simulink model "MotorModelZJChen"  (R2020b)
settings: Solver=VariableStepAuto  StartTime=0.0  StopTime=10.0  RelTol=1e-3  EnableMultiTasking=on
undefined symbols (not defined in the file): Aero, Initial, Motor, Uav
libraries: QuaternionLibrary x1
settings Model: Creator=jban039  LastModifiedBy=jban039
settings DataIOCC: LimitDataPoints=on
settings OptimizationCC: LifeSpan=inf
settings DebuggingCC: AllowSymbolicDim=off  SFUnexpectedBacktrackingDiag=warning  SFNoUnconditionalDefaultTransitionDiag=warning  SFExecutionAtInitializationDiag=none  ArithmeticOperatorsInVariantConditions=warning
settings ModelReferenceCC: PropagateSignalLabelsOutOfModel=off
settings SFSimCC: SimUseLocalCustomCode=off  CustomCodeUndefinedFunction=UseInterfaceOnly
settings RTWCC: RTWUseLocalCustomCode=off
settings CodeAppCC: StateflowObjectComments=on
settings GRTTargetCC: TargetLangStandard=C89/C90 (ANSI)
settings ConfigComp: CovMetricSettings=dw  CovSaveCumulativeToWorkspaceVar=on  CovSaveSingleToWorkspaceVar=on  CovExternalEMLEnable=off

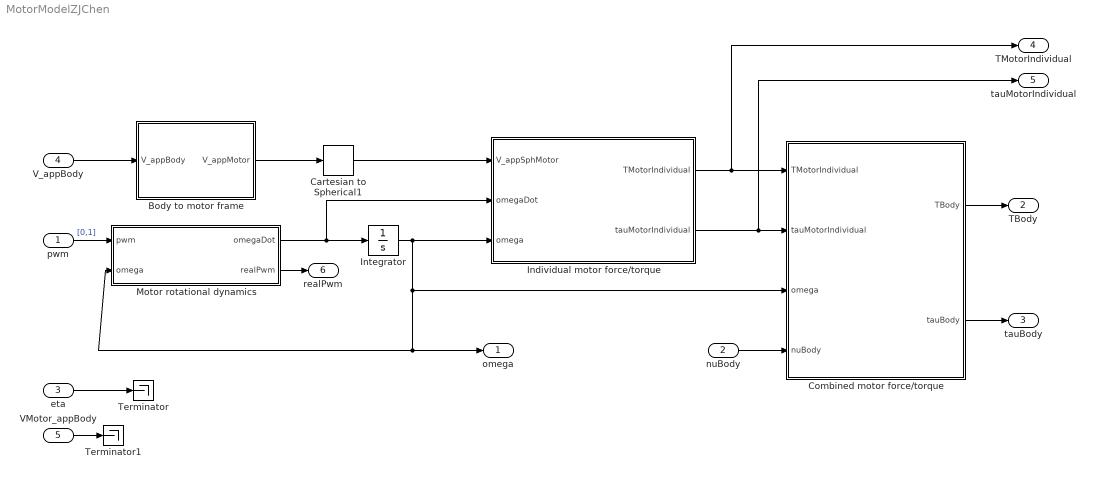
== system MotorModelZJChen ==
  pwm : Inport  PortDimensions=Uav.N_ROTORS
  nuBody : Inport  Port=2  Unit=rad/s  PortDimensions=3
  eta : Inport  Port=3  Unit=rad  PortDimensions=3
  V_appBody : Inport  Port=4  Unit=m/s  PortDimensions=3
  VMotor_appBody : Inport  Port=5  Unit=m/s  PortDimensions=[3,Uav.N_ROTORS]
  Body to motor frame : MATLAB Function  TreatAsAtomicUnit=on
  Cartesian to Spherical1 : QuaternionLibrary/Cartesian to Spherical
  Combined motor force/torque : MATLAB Function  TreatAsAtomicUnit=on
  Individual motor force/torque : MATLAB Function  TreatAsAtomicUnit=on
  Integrator : Integrator  InitialCondition=Initial.OMEGA  LimitOutput=on  LowerSaturationLimit=zeros(size(Initial.OMEGA))  ContinuousStateAttributes='omega'
  Motor rotational dynamics : MATLAB Function  TreatAsAtomicUnit=on
  Terminator : Terminator
  Terminator1 : Terminator
  omega : Outport  Unit=rad/s  VectorParamsAs1DForOutWhenUnconnected=off
  TBody : Outport  Port=2  Unit=N  VectorParamsAs1DForOutWhenUnconnected=off
  tauBody : Outport  Port=3  Unit=N*m  VectorParamsAs1DForOutWhenUnconnected=off
  TMotorIndividual : Outport  Port=4  Unit=N  PortDimensions=[3,Uav.N_ROTORS]  VectorParamsAs1DForOutWhenUnconnected=off
  tauMotorIndividual : Outport  Port=5  Unit=N  PortDimensions=[3,Uav.N_ROTORS]  VectorParamsAs1DForOutWhenUnconnected=off
  realPwm : Outport  Port=6  VectorParamsAs1DForOutWhenUnconnected=off
  wires:
  Combined motor force/torque/2(tauBody) -> tauBody/1
  Combined motor force/torque/1(TBody) -> TBody/1
  pwm/1 -> Motor rotational dynamics/1(pwm)  "[0,1]"
  eta/1 -> Terminator/1
  V_appBody/1 -> Body to motor frame/1(V_appBody)
  Individual motor force/torque/2(tauMotorIndividual) -> tauMotorIndividual/1, Combined motor force/torque/2(tauMotorIndividual)
  nuBody/1 -> Combined motor force/torque/4(nuBody)
  Individual motor force/torque/1(TMotorIndividual) -> TMotorIndividual/1, Combined motor force/torque/1(TMotorIndividual)
  Motor rotational dynamics/1(omegaDot) -> Individual motor force/torque/2(omegaDot), Integrator/1
  Integrator/1 -> Individual motor force/torque/3(omega), Combined motor force/torque/3(omega), Motor rotational dynamics/2(omega), omega/1
  Motor rotational dynamics/2(realPwm) -> realPwm/1
  VMotor_appBody/1 -> Terminator1/1
  Body to motor frame/1(V_appMotor) -> Cartesian to Spherical1/1
  Cartesian to Spherical1/1 -> Individual motor force/torque/1(V_appSphMotor)

== matlab function MotorModelZJChen/Body to motor frame ==
  data: V_appBody input; V_appMotor output; Uav parameter
function V_appMotor = BodyToMotor( V_appBody, Uav )
%#codegen
    V_appMotor = [Uav.GAMMA';Uav.GAMMA';Uav.GAMMA'] .* 0;
    for i = 1:Uav.N_ROTORS
        V_appMotor(:,i) = Uav.R_MOTOR_TO_BODY(:,:,i)' * V_appBody;
    end
end

== matlab function MotorModelZJChen/Individual motor force//torque ==
  data: V_appSphMotor input; omegaDot input; omega input; TMotorIndividual output; Motor parameter; Uav parameter; tauMotorIndividual output; Aero parameter
function [TMotorIndividual, tauMotorIndividual] = motorIndividual( ...
    V_appSphMotor, omegaDot, omega, Motor, Uav, Aero )
%#codegen
    alpha = V_appSphMotor(2,:);
    beta  = V_appSphMotor(1,:);
    U     = V_appSphMotor(3,:);
    
    % Make assertions to avoid code generation errors
    %assert(Uav.N_ROTORS < 16);

    %% Thrusts
    % Concatenated motor force/torque vectors in respective motor frame
    % eg. TMotor = [TMotor1, TMotor2, ..., TMotorN]
    % where: - N is the number of rotors
    %        - TMotorx (x ∈ [1,2,...,N]) is the thrust generated by motor x in
    %          its own frame of reference
    % For basic thrust model:
    % TMotorIndividual = [ zeros(2, Uav.N_ROTORS);
    %                      K * (omega'.^2) ];

    Cz2 = dot( Aero.Cz2.coefs*ones(size(alpha)), [alpha; ones(size(alpha))]);
    p = Aero.Cz3.coefs;
    lambda = omega' .* Uav.D_PROP ./ ( 2 .* U );
    Cz3 = p(1) * sin(alpha) + p(2) * ( 1 - exp(-p(3).*lambda) ) .* sin(3*alpha) + ...
        p(4);
    p = Aero.Cx2.coefs;
    Cx2 = p(1) * ( 1 - exp(-p(2).*lambda) ) .* cos(alpha) + ...
          p(3) * ( 1 - exp(-p(4).*lambda) ) .* cos(3*alpha);
    Tz = -0.5 .* Uav.RHO_AIR .* omega'.^2 .* (Cz2) .* Uav.D_PROP^2 .* Uav.A_PROP - ... % Rotor thrust
          0.5 .* Uav.RHO_AIR .* (Cz3) .* U .*  omega' .* Uav.D_PROP .* Uav.A_PROP;    % Rotor thrust correction
    Txy = -0.5 .* Uav.RHO_AIR .* (Cx2) .* U .* omega' .* Uav.D_PROP .* Uav.A_PROP;
    TMotorIndividual = [ Txy.*cos(beta); Txy.*sin(beta); Tz ];

    %% Moments
    p = Aero.CM2.coefs;
    CM2 = p(1) .* ( 1 - exp(-p(2).*lambda) ) .* cos(alpha) + ...
          p(3) .* ( 1 - exp(-p(4).*lambda) ) .* sin(2*alpha);
    Mxy = 0.5 .* Uav.RHO_AIR .* U .* omega' .* CM2 .* Uav.A_PROP .* Uav.D_PROP^2;
    % Avoid using zeros(1,Uav.N_ROTORS), which causes issues
    tauMotorIndividual = [ Mxy.*sin(beta); Mxy.*cos(beta);
        -Uav.ROTOR_DIRECTION .* ( Motor.C_TAU .* omega'.^2 + Motor.I_R_ZZ .* omegaDot' ) ];
end

== matlab function MotorModelZJChen/Motor rotational dynamics ==
  data: pwm input; omegaDot output; omega input; realPwm output; Motor parameter
function [omegaDot, realPwm]  = motorRotDynamics( pwm, omega, Motor )
%#codegen
%MOTORROTDYNAMICS Implement brushless DC motor model.
%   Based on permanent magnet DC motor model.
%   Written: J.X.J. Bannwarth

    % Normalised PWM (in [0, 1] range) to voltage conversion
    Vi = 6.9817.*pwm + 2.3508;

    % Motor dynamics
    omegaDot = (1./Motor.I_R_ZZ') .* ( ...
        (Motor.K_T/Motor.R) .* ( Vi - Motor.I_0*Motor.R - omega.*Motor.K_E ) - ...
        Motor.C_TAU.*omega.^2 );

    % Compute real PWM (in us) from normalised PWM
    realPwm = pwm.*(1950-1075) + 1075;
end

== matlab function MotorModelZJChen/Combined motor force//torque ==
  data: TMotorIndividual input; TBody output size=3; tauMotorIndividual input; tauBody output size=3; omega input; nuBody input; Motor parameter; Uav parameter
function [TBody, tauBody] = motorCombined( TMotorIndividual,tauMotorIndividual,  ...
    omega, nuBody, Motor, Uav)
%#codegen
assert(Uav.N_ROTORS < 16);

% Initialise matrices to store motor force/torque vectors in body frame
TBodyIndividual   = zeros(3, Uav.N_ROTORS);
tauBodyIndividual = zeros(3, Uav.N_ROTORS);

% Calculate forces and moments from each motor in the body frame
for i = 1:Uav.N_ROTORS
    l = Uav.L(i);
    gamma = Uav.GAMMA(i);
    
    % Matrix to compute torque applied by rotor thrust
 	L = [ 0,            0,            l*sin(gamma);
          0,            0,           -l*cos(gamma);
         -l*sin(gamma),  l*cos(gamma),  0 ];

	% Motor force/torque vectors in body frame
	TBodyIndividual(:,i) = Uav.R_MOTOR_TO_BODY(:,:,i) * ...
        TMotorIndividual(:,i);
	tauBodyIndividual(:,i) = Uav.R_MOTOR_TO_BODY(:,:,i) * ...
        tauMotorIndividual(:,i) + L * TBodyIndividual(:,i);
end

%% Gyroscopic moments

% Concatenated gyroscopic moments for each rotor
M_GBodyIndividual = zeros(3, Uav.N_ROTORS);
H_MMotorSeparate = zeros(3, Uav.N_ROTORS);

% Concatenated motor speeds in their respective frames
omegaMotor = [ zeros(2, Uav.N_ROTORS);
               Uav.ROTOR_DIRECTION .* omega' ];

for i = 1:Uav.N_ROTORS
    % Angular momentum in motor frame
    H_MMotorSeparate(:,i) = Motor.I_R(:,:,i) * omegaMotor(:,i);
    % Gyroscopic moment vectors in body frame
    M_GBodyIndividual(:,i) = cross( nuBody, ...
        Uav.R_MOTOR_TO_BODY(:,:,i) * H_MMotorSeparate(:,i) );
end

M_GBody = sum(M_GBodyIndividual, 2);

%% Total torque and moment

% Total force/torque in body frame
TBody = sum(TBodyIndividual, 2);
tauBody = sum(tauBodyIndividual, 2) - M_GBody;

end
